simulink model "fxpdemo_dtprop"  (Simulink 5.0)
settings: Solver=FixedStepDiscrete  StartTime=0.0  StopTime=10.0  FixedStep=0.01  RelTol=1e-3
libraries: fixpt_dtprop x6, fixpt_lib_4 x6
settings Model: CovMetricSettings=d  MinMaxOverflowLogging=MinMaxAndOverflow  Creator=andyb  LastModifiedBy=andyb  ExtModeAutoUpdateStatusClock=off  ParameterDowncastMsg=warning  ParameterOverflowMsg=warning  ParameterPrecisionLossMsg=none  BlockReductionOpt=off  BooleanDataType=off

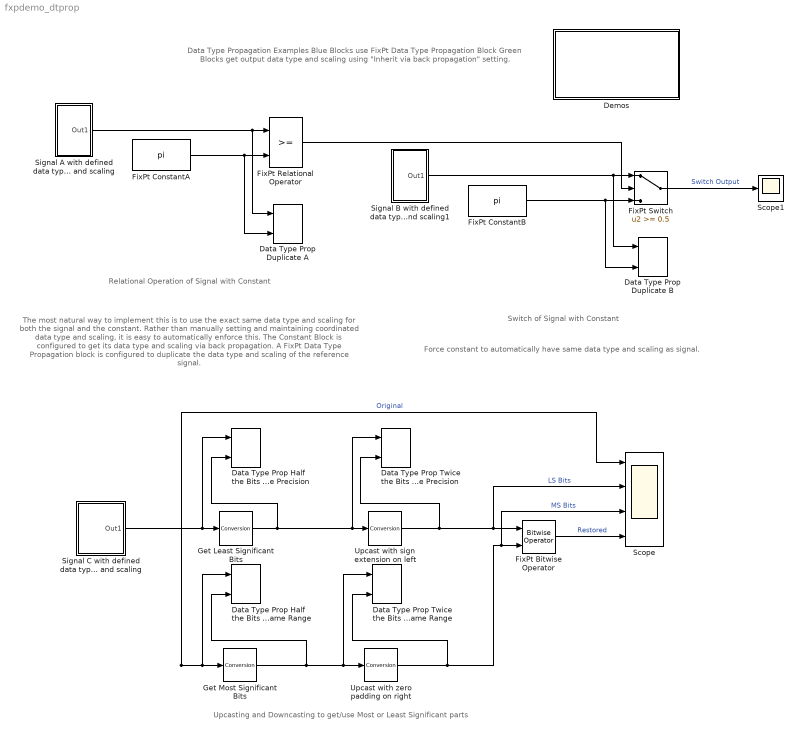
== system fxpdemo_dtprop ==
  note: The most natural way to implement this is to use the exact same
      | data type and scaling for both the signal and the constant.  Rather
      | than manually setting and maintaining coordinated data type and
      | scaling, it is easy to automatically enforce this.  The Constant Block
      | is configured to get its data type and scaling via back propagation.
      | A FixPt Data Type Propagation block is configured to duplicate the
      | data type and scaling of the reference signal.
  note: Relational Operation of Signal with Constant
  note: Force constant to automatically have same
      | data type and scaling as signal.
  note: Switch of Signal with Constant
  note: Data Type Propagation Examples
      |
      | Blue Blocks use FixPt Data Type Propagation Block
      |
      | Green Blocks get output data type and scaling using
      | "Inherit via back propagation" setting.
  note: Upcasting and Downcasting to get/use Most or Least Significant parts
  Data Type Prop Duplicate A : fixpt_dtprop/Data Type Prop Duplicate  SimViewingDevice=off  DataTypeOverride=UseLocalSettings  MinMaxOverflowLogging=UseLocalSettings
      settings: Permissions=ReadWrite  RTWFcnNameOpts=Auto  RTWFileNameOpts=Auto
  Data Type Prop Duplicate B : fixpt_dtprop/Data Type Prop Duplicate  SimViewingDevice=off  DataTypeOverride=UseLocalSettings  MinMaxOverflowLogging=UseLocalSettings
      settings: Permissions=ReadWrite  RTWFcnNameOpts=Auto  RTWFileNameOpts=Auto
  Data Type Prop Half the Bits Same Precision : fixpt_dtprop/Data Type Prop Half the Bits Same Precision  SimViewingDevice=off  DataTypeOverride=UseLocalSettings  MinMaxOverflowLogging=UseLocalSettings
      settings: Permissions=ReadWrite  RTWFcnNameOpts=Auto  RTWFileNameOpts=Auto
  Data Type Prop Half the Bits Same Range : fixpt_dtprop/Data Type Prop Half the Bits Same Range  SimViewingDevice=off  DataTypeOverride=UseLocalSettings  MinMaxOverflowLogging=UseLocalSettings
      settings: Permissions=ReadWrite  RTWFcnNameOpts=Auto  RTWFileNameOpts=Auto
  Data Type Prop Twice the Bits Same Precision : fixpt_dtprop/Data Type Prop Twice the Bits Same Precision  SimViewingDevice=off  DataTypeOverride=UseLocalSettings  MinMaxOverflowLogging=UseLocalSettings
      settings: Permissions=ReadWrite  RTWFcnNameOpts=Auto  RTWFileNameOpts=Auto
  Data Type Prop Twice the Bits Same Range : fixpt_dtprop/Data Type Prop Twice the Bits Same Range  SimViewingDevice=off  DataTypeOverride=UseLocalSettings  MinMaxOverflowLogging=UseLocalSettings
      settings: Permissions=ReadWrite  RTWFcnNameOpts=Auto  RTWFileNameOpts=Auto
  Demos : Subsystem
      settings: OpenFcn=open_system('fixpt_dtprop')
      mask Display: disp('Go to Library with\nExample Uses of\nData Type\nPropagation Block')
  FixPt Bitwise Operator : fixpt_lib_4/Bits/Bitwise Operator  logicop=OR  UseBitMask=off  NumInputPorts=2  BitMask=2^5+2^2+2^0  BitMaskRealWorld=Stored Integer
  FixPt ConstantA : Constant  Value=pi  ShowAdditionalParam=on  OutDataType=ufix(16)  OutScaling=2^-12
  FixPt ConstantB : Constant  Value=pi  ShowAdditionalParam=on  OutDataType=ufix(16)  OutScaling=2^-12
  FixPt Relational Operator : RelationalOperator  ShowAdditionalParam=on  LogicOutDataTypeMode=Specify via dialog
  FixPt Switch : Switch  Threshold=0.5  ShowAdditionalParam=on
  Get Least Significant Bits : fixpt_lib_4/Data Type/Conversion  ConvertRealWorld=Real World Value  OutDataType=sfix(16)  OutScaling=2^-10  DoSatur=off
  Get Most Significant Bits : fixpt_lib_4/Data Type/Conversion  ConvertRealWorld=Real World Value  OutDataType=sfix(16)  OutScaling=2^-10  DoSatur=off
  Scope : Scope  NumInputPorts=4
      settings: TimeRange=10  YMin=500~-5~-5~-5  YMax=1500~5~5~5
  Scope1 : Scope
      settings: TimeRange=10  YMin=370  YMax=405
  Signal A with defined data type and scaling : Subsystem
  Signal B with defined data type and scaling1 : Subsystem
  Signal C with defined data type and scaling : Subsystem
  Upcast with sign extension on left : fixpt_lib_4/Data Type/Conversion  ConvertRealWorld=Real World Value  OutDataType=sfix(16)  OutScaling=2^-10  DoSatur=off
  Upcast with zero padding on right : fixpt_lib_4/Data Type/Conversion  ConvertRealWorld=Real World Value  OutDataType=sfix(16)  OutScaling=2^-10  DoSatur=off
  wires:
  Signal A with defined data type and scaling/1(Out1) -> FixPt Relational Operator/1, Data Type Prop Duplicate A/1
  FixPt ConstantA/1 -> FixPt Relational Operator/2, Data Type Prop Duplicate A/2
  FixPt Relational Operator/1 -> FixPt Switch/2
  Signal B with defined data type and scaling1/1(Out1) -> Data Type Prop Duplicate B/1, FixPt Switch/1
  FixPt ConstantB/1 -> Data Type Prop Duplicate B/2, FixPt Switch/3
  FixPt Switch/1 -> Scope1/1  "Switch Output"
  Signal C with defined data type and scaling/1(Out1) -> Get Least Significant Bits/1, Data Type Prop Half the Bits Same Precision/1, Data Type Prop Half the Bits Same Range/1, Get Most Significant Bits/1, Scope/1  "Original"
  Get Least Significant Bits/1 -> Data Type Prop Half the Bits Same Precision/2, Data Type Prop Twice the Bits Same Precision/1, Upcast with sign extension on left/1
  Get Most Significant Bits/1 -> Data Type Prop Half the Bits Same Range/2, Upcast with zero padding on right/1, Data Type Prop Twice the Bits Same Range/1
  Upcast with sign extension on left/1 -> Data Type Prop Twice the Bits Same Precision/2, FixPt Bitwise Operator/1, Scope/2  "LS Bits"
  Upcast with zero padding on right/1 -> Data Type Prop Twice the Bits Same Range/2, FixPt Bitwise Operator/2, Scope/3  "MS Bits"
  FixPt Bitwise Operator/1 -> Scope/4  "Restored"

== system fxpdemo_dtprop/Demos ==

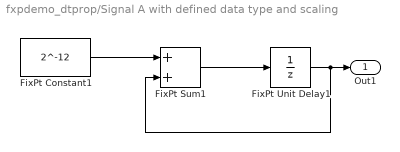
== system fxpdemo_dtprop/Signal A with defined data type and scaling ==
  FixPt Constant1 : Constant  Value=2^-12  ShowAdditionalParam=on  OutDataTypeMode=Specify via dialog  OutScaling=2^-12
  FixPt Sum1 : Sum  ShowAdditionalParam=on  OutDataType=ufix(16)  OutScaling=[2^-12]
  FixPt Unit Delay1 : UnitDelay  X0=3  SampleTime=-1
  Out1 : Outport
  wires:
  FixPt Constant1/1 -> FixPt Sum1/1
  FixPt Sum1/1 -> FixPt Unit Delay1/1
  FixPt Unit Delay1/1 -> FixPt Sum1/2, Out1/1

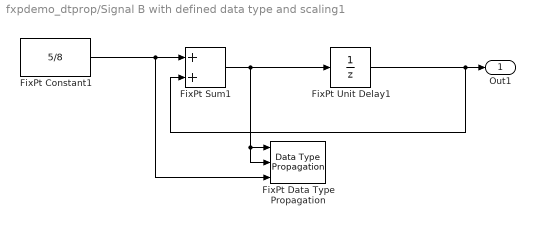
== system fxpdemo_dtprop/Signal B with defined data type and scaling1 ==
  FixPt Constant1 : Constant  Value=5/8  ShowAdditionalParam=on  OutDataType=ufix(8)  OutScaling=[5/8 371]
  FixPt Data Type Propagation : fixpt_lib_4/Data Type/Data Type Propagation  PropDataType=sfix(16)  IfRefDouble=double  IfRefSingle=single  IsSigned=IsSigned1  NumBitsBase=NumBits1  NumBitsMult=1  NumBitsAdd=0  NumBitsAllowFinal=1:128  PropScaling=2^-10  ValuesUsedBestPrec=[5 -7]  SlopeBase=Slope1  SlopeMult=1  SlopeAdd=0  BiasBase=Bias1  BiasMult=0  BiasAdd=0
  FixPt Sum1 : Sum  ShowAdditionalParam=on  OutDataTypeMode=Specify via dialog  OutDataType=ufix(8)  OutScaling=[5/8 371]
  FixPt Unit Delay1 : UnitDelay  SampleTime=-1
  Out1 : Outport
  wires:
  FixPt Unit Delay1/1 -> Out1/1, FixPt Sum1/2
  FixPt Sum1/1 -> FixPt Unit Delay1/1, FixPt Data Type Propagation/2, FixPt Data Type Propagation/1
  FixPt Constant1/1 -> FixPt Sum1/1, FixPt Data Type Propagation/3

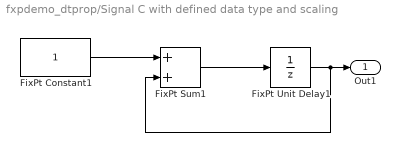
== system fxpdemo_dtprop/Signal C with defined data type and scaling ==
  FixPt Constant1 : Constant  ShowAdditionalParam=on  OutDataTypeMode=Specify via dialog  OutDataType=ufix(16)
  FixPt Sum1 : Sum  ShowAdditionalParam=on  OutDataType=ufix(16)  OutScaling=[2^-12]
  FixPt Unit Delay1 : UnitDelay  X0=500  SampleTime=-1
  Out1 : Outport
  wires:
  FixPt Unit Delay1/1 -> Out1/1, FixPt Sum1/2
  FixPt Sum1/1 -> FixPt Unit Delay1/1
  FixPt Constant1/1 -> FixPt Sum1/1
